simulink model "TS1_Version_1_ohne_Edge_detector"  (R2012b)
settings: Solver=FixedStepDiscrete  StartTime=0.0  StopTime=100  RelTol=1e-3
libraries: c2833xlib x2, idelinklib_tgtpref x1, c280xlib x1
settings Model: Creator=Nikolay  LastModifiedBy=Nikolay
settings DataIOCC: SaveOutput=off  SaveTime=off
settings OptimizationCC: OptimizeModelRefInitCode=on  LifeSpan=1
settings HardwareCC: ProdBitPerChar=16  ProdBitPerInt=16  ProdBitPerPointer=16  ProdLargestAtomicInteger=Integer  ProdIntDivRoundTo=Zero  ProdEndianess=LittleEndian  ProdWordSize=16  ProdHWDeviceType=Texas Instruments->C2000
settings RTWCC: SystemTargetFile=idelink_ert.tlc  GenerateMakefile=off  TemplateMakefile=none  Description=IDE Link ERT  ProcessScript=idelink_ert_make_rtw_hook
settings CodeAppCC: IgnoreCustomStorageClasses=off

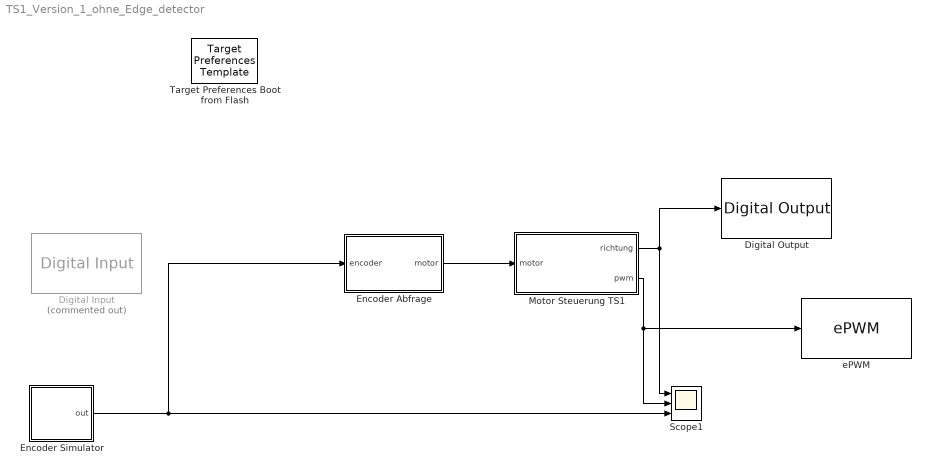
== system TS1_Version_1_ohne_Edge_detector ==
  Digital Input : c2833xlib/Digital Input  Commented=on  GPIO_Number=GPIO24~GPIO31  GPIO_Bit0=on  GPIO_Bit1=off  GPIO_Bit2=off  GPIO_Bit3=off  GPIO_Bit4=off  GPIO_Bit5=off  GPIO_Bit6=off  GPIO_Bit7=off  sampleTime=0.00001  dataType=auto  GPIO_Bit0_Qualification=Sync to SYSCLKOUT  GPIO_Bit1_Qualification=Sync to SYSCLKOUT  GPIO_Bit2_Qualification=Sync to SYSCLKOUT  GPIO_Bit3_Qualification=Sync to SYSCLKOUT  GPIO_Bit4_Qualification=Sync to SYSCLKOUT  GPIO_Bit5_Qualification=Sync to SYSCLKOUT  GPIO_Bit6_Qualification=Sync to SYSCLKOUT  GPIO_Bit7_Qualification=Sync to SYSCLKOUT  Qualification_Period=-1
  Digital Output : c2833xlib/Digital Output  GPIO_Number=GPIO16~GPIO23  GPIO_Bit0=off  GPIO_BIT0_Toggle=off  GPIO_Bit1=off  GPIO_BIT1_Toggle=off  GPIO_Bit2=off  GPIO_BIT2_Toggle=off  GPIO_Bit3=off  GPIO_BIT3_Toggle=off  GPIO_Bit4=off  GPIO_BIT4_Toggle=off  GPIO_Bit5=on  GPIO_BIT5_Toggle=off  GPIO_Bit6=off  GPIO_BIT6_Toggle=off  GPIO_Bit7=off  GPIO_BIT7_Toggle=off
  Encoder Abfrage : Stateflow chart  TreatAsAtomicUnit=on
  Encoder Simulator : Stateflow chart  TreatAsAtomicUnit=on
  Motor Steuerung TS1 : Stateflow chart  TreatAsAtomicUnit=on
  Scope1 : Scope  NumInputPorts=3
      settings: YMin=-5~-5~-5  YMax=5~5~5
  Target Preferences Boot from Flash : idelinklib_tgtpref/Target Preferences Template  Tag=ccslinktgtpref_ccsv4  library=off
  ePWM : c280xlib/ePWM  checkMode=off  useModule=ePWM2  periodUnits=Clock cycles  timerSource=Specify via dialog  timerPeriod_clk=64000  timerPeriod_sec=0.0001  countingMode=Up  synchronizationOption=Disable  synchronizationEnable=off  phaseActiveEnable=Disable  phaseDirection=Count down after sync  phaseActive=0  clockPrescale=1  HSclockPrescale=1  ePWMxAStatus=on  CMPAUnits=Clock cycles  CMPASource=Specify via dialog  CMPAValue_per=50  CMPAValue_clk=32000  ePWMxAactionLogic1=Do nothing  ePWMxAactionLogic2=Clear  ePWMxAactionLogic3=Set  ePWMxAactionLogic4=Do nothing  ePWMxAactionLogic5=Do nothing  ePWMxAactionLogic6=Do nothing  ePWMxALoadMode=Load on CTR=Zero  ePWMxACSFenable=off  ePWMxACSFvalue=Forcing Disable  ePWMxASFreload=Zero  enHRPWM=off  HRPWM_LoadMode=CTR=ZERO  HRPWM_CTLMode=Phase control mode  HRPWM_EDGMode=Both edge  enSFO=on  ePWMxBStatus=on  CMPBUnits=Percentages  CMPBSource=Input port  CMPBValue_per=0  CMPBValue_clk=0  ePWMxBactionLogic1=Do nothing  ePWMxBactionLogic2=Set  ePWMxBactionLogic3=Do nothing  ePWMxBactionLogic4=Do nothing  ePWMxBactionLogic5=Clear  ePWMxBactionLogic6=Do nothing  ePWMxBLoadMode=Load on CTR=Zero  ePWMxBCSFenable=off  ePWMxBCSFvalue=Forcing Disable  ePWMxBSFreload=Zero  enableDBePWMxA=off  enableDBePWMxB=off  DBpolarity=AH  DBedgeDelay=Positive  DBSource_ePWMxA=ePWMxA  DBSource_ePWMxB=ePWMxA  DBperiodSource=Specify via dialog  REDperiod=0  FEDperiod=0  adcstartModuleA=off  adcrequestEventA=First event  adcstartEventA=CTR=Zero  adcstartModuleB=off  adcrequestEventB=First event  adcstartEventB=CTR=Zero  intEn=off  intPrd=First event  intSel=CTR=Zero  chopperEnable=off  chopperFrequency=1  chopperFirstwidth=1  chopperDuty=12.5%  tripZonesource=Specify via dialog  tzselOSHT1=off  tzselOSHT2=off  tzselOSHT3=off  tzselOSHT4=off  tzselOSHT5=off  tzselOSHT6=off  tzselCBC1=off  tzselCBC2=off  tzselCBC3=off  tzselCBC4=off  tzselCBC5=off  tzselCBC6=off  enTzOstIntr=off  enTzCbcIntr=off  ePWMxAforced=No action  ePWMxBforced=No action  timerPeriod=-1  ePWMxAValue=0  ePWMxBValue=0  tripZoneoption=OSHT
  wires:
  Motor Steuerung TS1/2(pwm) -> ePWM/1, Scope1/2
  Motor Steuerung TS1/1(richtung) -> Digital Output/1, Scope1/1
  Encoder Simulator/1(out) -> Encoder Abfrage/1(encoder), Scope1/3
  Encoder Abfrage/1(motor) -> Motor Steuerung TS1/1(motor)

== stateflow chart TS1_Version_1_ohne_Edge_detector/Motor Steuerung TS1 ==
  note: # Richtungsvariable: 0 - nach vorne, 1 - nach hinten
      | # Motorvariable: 0 - gesperrt, 1 - funktioniert
      | # PWM Wert im Normalbetrieb muss heueristisch bestimmt werden (einfach Testen)
  state Start
    pwm = 60;
    richtung = 0;
  state Normalbetrieb
    richtung = 0;
    pwm = 60;
  state Abfrage
    motor;
  note: # Wartezeit muss auch wie PWM bestimmt werden
  state PWM_increment
    pwm =pwm+10
  note: # Wartezeit muss auch wie PWM bestimmt werden
  state Rueckfahrt
    pwm= 80;
    richtung = 1;
  (default) -> Start
  Rueckfahrt -> Start : [ after(2,sec)]
  Start -> Abfrage
  Normalbetrieb -> Abfrage
  Abfrage -> Normalbetrieb [order 2] : [motor == 1]
  PWM_increment -> Abfrage [order 1] : [pwm!= 100]
  Abfrage -> PWM_increment [order 1] : [after(1,sec) && motor == 0]
  PWM_increment -> Rueckfahrt [order 2] : [pwm == 100]
  data: motor input; richtung output double; pwm output double

== stateflow chart TS1_Version_1_ohne_Edge_detector/Encoder Abfrage ==
  state Start
    motor = 1;
  state Zwischenschritt
  note: # Wartezeit muss auch wie PWM bestimmt werden
  state Abfrage_laufen
    encoder;
  state Ausgabe_laufend
    motor =1;
  state Ausgabe_gesperrt
    motor =0;
  (default) -> Start
  Start -> Zwischenschritt
  Ausgabe_gesperrt -> Zwischenschritt
  Ausgabe_laufend -> Zwischenschritt
  Zwischenschritt -> Abfrage_laufen : [after(2,sec)]
  Abfrage_laufen -> Ausgabe_laufend [order 2] : [after(1,sec) && encoder == 1 ]
  Abfrage_laufen -> Ausgabe_gesperrt [order 1] : [after(1,sec) && encoder == 0 ]
  data: encoder input; motor output double

== stateflow chart TS1_Version_1_ohne_Edge_detector/Encoder Simulator ==
  state Start
    out = 8
    counter = 0
  state High
    out = 8
    counter = counter +1
  state Low
    out = 0
  state Wieder_Gesperrt
    out = 8
  (default) -> Start
  Start -> High : [after(20,sec)]
  High -> Low [order 1] : [after(1,sec) && counter <= 10]
  Low -> High : [after(1,sec) && counter <= 10]
  High -> Wieder_Gesperrt [order 2] : [counter > 10]
  data: out output double; counter local double
